simulink model "gradients_simu_v1"  (R2020b)
settings: Solver=FixedStepDiscrete  StartTime=0.0  StopTime=simTime  RelTol=1e-3
InitFcn:
  | generate_locals_for_simulink
undefined symbols (not defined in the file): gray, Hg
libraries: simulink x6, visionhdlio x3, visionhdlutilities x2, visionstatistics x1, visionhdlfilter x1, dspvision x1
settings Model: DataTypeOverride=Off  SimulationMode=accelerator  Creator=The MathWorks, Inc.  LastModifiedBy=Ethan
settings SolverCC: AutoInsertRateTranBlk=on
settings DataIOCC: LimitDataPoints=on  SaveOutput=off  SignalLogging=off  SaveTime=off  ReturnWorkspaceOutputs=off
settings OptimizationCC: BlockReduction=off  ConditionallyExecuteInputs=off  DefaultParameterBehavior=Inlined  LifeSpan=inf
settings DebuggingCC: AlgebraicLoopMsg=error  SingleTaskRateTransMsg=error  ParameterPrecisionLossMsg=none  AllowSymbolicDim=off  StrictBusMsg=ErrorOnBusTreatedAsVector  SFUnexpectedBacktrackingDiag=warning  SFNoUnconditionalDefaultTransitionDiag=warning  SFExecutionAtInitializationDiag=none  ArithmeticOperatorsInVariantConditions=warning
settings HardwareCC: ProdBitPerPointer=32  ProdBitPerSizeT=32  ProdBitPerPtrDiffT=32  ProdLargestAtomicFloat=None  ProdIntDivRoundTo=Undefined  ProdEndianess=Unspecified  ProdWordSize=32  ProdHWDeviceType=ASIC/FPGA->ASIC/FPGA  ProdEqTarget=off
settings SFSimCC: SimUseLocalCustomCode=off  CustomCodeUndefinedFunction=UseInterfaceOnly
settings RTWCC: RTWUseLocalCustomCode=off
settings CodeAppCC: StateflowObjectComments=on
settings GRTTargetCC: TargetLangStandard=C89/C90 (ANSI)
settings ConfigComp: CovMetricSettings=dw  CovSaveCumulativeToWorkspaceVar=on  CovSaveSingleToWorkspaceVar=on  CovExternalEMLEnable=off  CovSFcnEnable=off

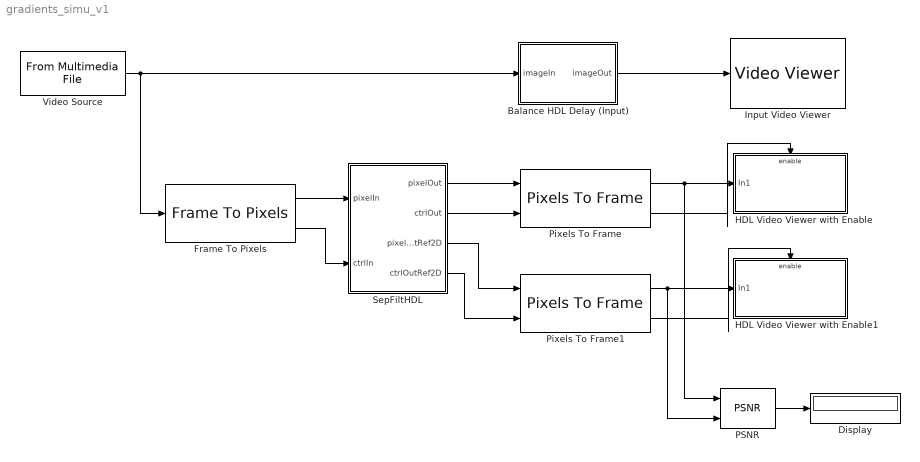
== system gradients_simu_v1 ==
  Balance HDL Delay (Input) : Subsystem
  Display : Display
  Frame To Pixels : visionhdlio/Frame To Pixels  NumComponents=1  NumPixels=1  VideoFormat=480p  ActivePixelsPerLine=32  ActiveVideoLines=18  TotalPixelsPerLine=42  TotalVideoLines=28  StartingActiveLine=6  FrontPorch=5  SampleTime=0
      settings: SourceProductName=Vision HDL Toolbox
  HDL Video Viewer with Enable : Subsystem
  HDL Video Viewer with Enable1 : Subsystem
  Input Video Viewer : VideoViewer  colormapValue=gray(256)  FigPos=[27 749 754 601]
  PSNR : visionstatistics/PSNR
      settings: SourceProductName=Computer Vision Toolbox
  Pixels To Frame : visionhdlio/Pixels To Frame  NumComponents=1  NumPixels=1  VideoFormat=480p  ActivePixelsPerLine=32  ActiveVideoLines=18  TotalPixelsPerLine=42  TotalVideoLines=28
      settings: SourceProductName=Vision HDL Toolbox
  Pixels To Frame1 : visionhdlio/Pixels To Frame  NumComponents=1  NumPixels=1  VideoFormat=480p  ActivePixelsPerLine=32  ActiveVideoLines=18  TotalPixelsPerLine=42  TotalVideoLines=28
      settings: SourceProductName=Vision HDL Toolbox
  SepFiltHDL : Subsystem
  Video Source : dspvision/From Multimedia File  inputFilename=C:\Users\Ethan\Ravven_Labs_Ethan\ravven-tag\simulink\gradients\images\start.mp4  readRange=[1 Inf]  loop=on  numPlays=inf  outputStreams=Video only  videoDataType=uint8  audioDataType=int16  inheritSampleTime=off  userDefinedSampleTime=totalPixels  noAudioOutput=off  isIntensityVideo=off  fourcc=Intensity  colorVideoFormat=One multidimensional signal  outputEOF=off  dataOrg=Column-major  audioFrameSize=1024  computeAudioFrameSize=off  outSamplingMode=Sample based
  wires:
  Frame To Pixels/1 -> SepFiltHDL/1(pixelIn)
  SepFiltHDL/1(pixelOut) -> Pixels To Frame/1
  SepFiltHDL/2(ctrlOut) -> Pixels To Frame/2
  Video Source/1 -> Frame To Pixels/1, Balance HDL Delay (Input)/1(imageIn)
  Balance HDL Delay (Input)/1(imageOut) -> Input Video Viewer/1
  Pixels To Frame/1 -> PSNR/1, HDL Video Viewer with Enable/1(In1)
  Pixels To Frame1/2 -> HDL Video Viewer with Enable1/Enable
  SepFiltHDL/3(pixelOutRef2D) -> Pixels To Frame1/1
  SepFiltHDL/4(ctrlOutRef2D) -> Pixels To Frame1/2
  Frame To Pixels/2 -> SepFiltHDL/2(ctrlIn)
  Pixels To Frame/2 -> HDL Video Viewer with Enable/Enable
  Pixels To Frame1/1 -> PSNR/2, HDL Video Viewer with Enable1/1(In1)
  PSNR/1 -> Display/1

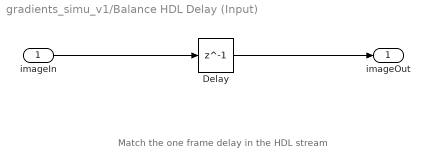
== system gradients_simu_v1/Balance HDL Delay (Input) ==
  note: Match the one frame delay in the HDL stream
  imageIn : Inport
  Delay : Delay  DelayLength=1
  imageOut : Outport  VectorParamsAs1DForOutWhenUnconnected=off
  wires:
  imageIn/1 -> Delay/1
  Delay/1 -> imageOut/1

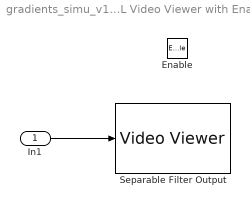
== system gradients_simu_v1/HDL Video Viewer with Enable ==
  In1 : Inport
  Enable : EnablePort
  Separable Filter Output : VideoViewer  colormapValue=gray(256)  FigPos=[579 975 702 585]
  wires:
  In1/1 -> Separable Filter Output/1

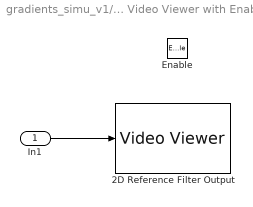
== system gradients_simu_v1/HDL Video Viewer with Enable1 ==
  In1 : Inport
  Enable : EnablePort
  2D Reference Filter Output : VideoViewer  colormapValue=gray(256)  FigPos=[1227 697 653 551]
  wires:
  In1/1 -> 2D Reference Filter Output/1

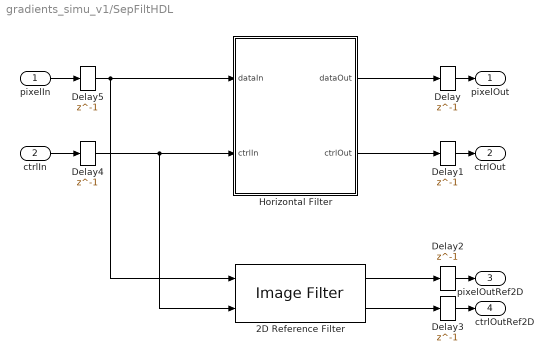
== system gradients_simu_v1/SepFiltHDL ==
  pixelIn : Inport
  ctrlIn : Inport  Port=2
  2D Reference Filter : visionhdlfilter/Image Filter  CoefficientsSource=Property  Coefficients=Hg  PaddingMethod=Constant  PaddingValue=0  LineBufferSize=2048  SimulateUsing=Code generation  roundingMode=Nearest  overflowMode=on  CoeffDataTypeStr=good_fixdt_hg  CoeffMin=[]  CoeffMax=[]  OutputMin=[]  OutputMax=[]
      settings: SourceProductName=Vision HDL Toolbox
  Delay{,1..5} (6 alike) : Delay  DelayLength=1
  Horizontal Filter : Subsystem
  pixelOut : Outport  VectorParamsAs1DForOutWhenUnconnected=off
  ctrlOut : Outport  Port=2  VectorParamsAs1DForOutWhenUnconnected=off
  pixelOutRef2D : Outport  Port=3  VectorParamsAs1DForOutWhenUnconnected=off
  ctrlOutRef2D : Outport  Port=4  VectorParamsAs1DForOutWhenUnconnected=off
  wires:
  ctrlIn/1 -> Delay4/1
  pixelIn/1 -> Delay5/1
  2D Reference Filter/2 -> Delay3/1
  2D Reference Filter/1 -> Delay2/1
  Horizontal Filter/1(dataOut) -> Delay/1
  Horizontal Filter/2(ctrlOut) -> Delay1/1
  Delay/1 -> pixelOut/1
  Delay1/1 -> ctrlOut/1
  Delay2/1 -> pixelOutRef2D/1
  Delay3/1 -> ctrlOutRef2D/1
  Delay4/1 -> Horizontal Filter/2(ctrlIn), 2D Reference Filter/2
  Delay5/1 -> Horizontal Filter/1(dataIn), 2D Reference Filter/1

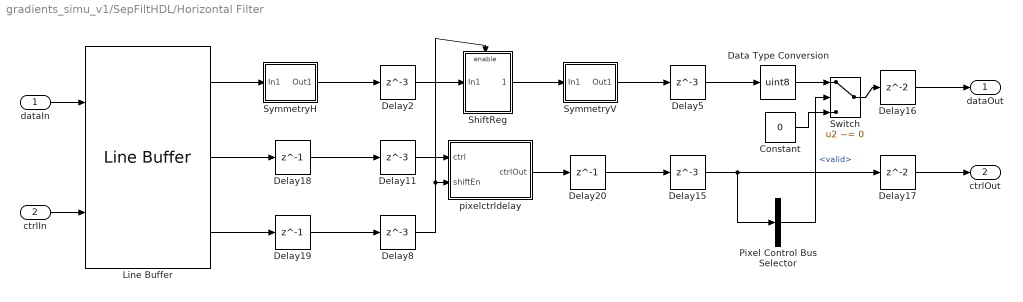
== system gradients_simu_v1/SepFiltHDL/Horizontal Filter ==
  dataIn : Inport
  ctrlIn : Inport  Port=2
  Constant : Constant  Value=0  OutDataTypeStr=Inherit: Inherit via back propagation  SampleTime=-1
  Data Type Conversion : DataTypeConversion  OutDataTypeStr=uint8  RndMeth=Nearest  SaturateOnIntegerOverflow=on
  Delay{2,5,8,11,15} (5 alike) : Delay  DelayLength=3
  Delay16 : Delay
  Delay17 : Delay
  Delay18 : Delay  DelayLength=1
  Delay19 : Delay  DelayLength=1
  Delay20 : Delay  DelayLength=1
  Line Buffer : visionhdlutilities/Line Buffer  NeighborhoodSize=[3 3]  PaddingMethod=Constant  PaddingValue=0  LineBufferSize=2048  SimulateUsing=Code generation
      settings: SourceProductName=Vision HDL Toolbox
  Pixel Control Bus Selector : BusSelector  OutputSignals=valid
  ShiftReg : Subsystem
  Switch : Switch  Criteria=u2 ~= 0
  SymmetryH : Subsystem
  SymmetryV : Subsystem
  pixelctrldelay : Subsystem
  dataOut : Outport  VectorParamsAs1DForOutWhenUnconnected=off
  ctrlOut : Outport  Port=2  VectorParamsAs1DForOutWhenUnconnected=off
  wires:
  Delay8/1 -> pixelctrldelay/2(shiftEn), ShiftReg/Enable
  SymmetryH/1(Out1) -> Delay2/1
  SymmetryV/1(Out1) -> Delay5/1
  Delay5/1 -> Data Type Conversion/1
  dataIn/1 -> Line Buffer/1
  Data Type Conversion/1 -> Switch/1
  Delay17/1 -> ctrlOut/1
  Constant/1 -> Switch/3
  Delay2/1 -> ShiftReg/1(In1)
  Switch/1 -> Delay16/1
  Delay15/1 -> Delay17/1, Pixel Control Bus Selector/1
  Pixel Control Bus Selector/1 -> Switch/2  "<valid>"
  ctrlIn/1 -> Line Buffer/2
  Delay16/1 -> dataOut/1
  Line Buffer/3 -> Delay19/1
  Line Buffer/2 -> Delay18/1
  ShiftReg/1(Out1) -> SymmetryV/1(In1)
  Line Buffer/1 -> SymmetryH/1(In1)
  Delay18/1 -> Delay11/1
  Delay19/1 -> Delay8/1
  Delay20/1 -> Delay15/1
  Delay11/1 -> pixelctrldelay/1(ctrl)
  pixelctrldelay/1(ctrlOut) -> Delay20/1

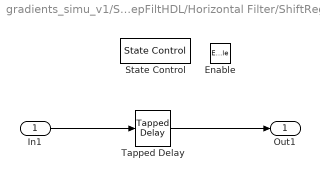
== system gradients_simu_v1/SepFiltHDL/Horizontal Filter/ShiftReg ==
  In1 : Inport
  Enable : EnablePort
  State Control : StateControl  StateControl=Synchronous
  Tapped Delay : simulink/Discrete/Tapped Delay  vinit=0.0  samptime=-1  NumDelays=3  DelayOrder=Oldest  includeCurrent=off
  Out1 : Outport  VectorParamsAs1DForOutWhenUnconnected=off
  wires:
  In1/1 -> Tapped Delay/1
  Tapped Delay/1 -> Out1/1

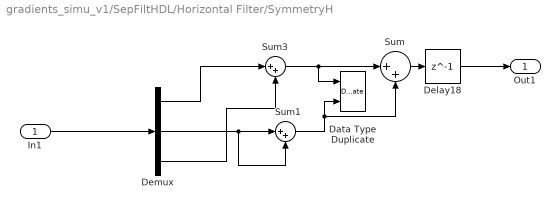
== system gradients_simu_v1/SepFiltHDL/Horizontal Filter/SymmetryH ==
  In1 : Inport
  Data Type Duplicate : DataTypeDuplicate
  Delay18 : Delay  DelayLength=1
  Demux : Demux  Outputs=3
  Sum : Sum  Inputs=|++
  Sum1 : Sum  Inputs=|++
  Sum3 : Sum  Inputs=|++
  Out1 : Outport  VectorParamsAs1DForOutWhenUnconnected=off
  wires:
  Sum3/1 -> Sum/1, Data Type Duplicate/1
  Sum1/1 -> Sum/2, Data Type Duplicate/2
  Delay18/1 -> Out1/1
  In1/1 -> Demux/1
  Demux/1 -> Sum3/1
  Demux/3 -> Sum3/2
  Demux/2 -> Sum1/2, Sum1/1
  Sum/1 -> Delay18/1

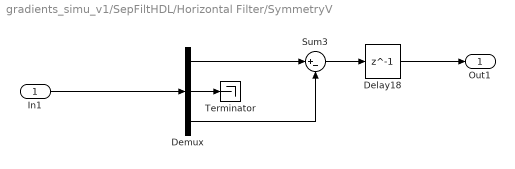
== system gradients_simu_v1/SepFiltHDL/Horizontal Filter/SymmetryV ==
  In1 : Inport
  Delay18 : Delay  DelayLength=1
  Demux : Demux  Outputs=3
  Sum3 : Sum  Inputs=|+-
  Terminator : Terminator
  Out1 : Outport  VectorParamsAs1DForOutWhenUnconnected=off
  wires:
  In1/1 -> Demux/1
  Delay18/1 -> Out1/1
  Demux/3 -> Sum3/2
  Demux/1 -> Sum3/1
  Demux/2 -> Terminator/1
  Sum3/1 -> Delay18/1

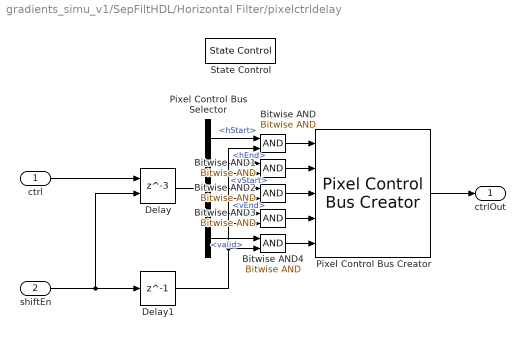
== system gradients_simu_v1/SepFiltHDL/Horizontal Filter/pixelctrldelay ==
  ctrl : Inport
  shiftEn : Inport  Port=2
  Bitwise AND{,1..4} (5 alike) : simulink/Logic and Bit Operations/Bitwise Operator  logicop=AND  UseBitMask=off  NumInputPorts=2  BitMask=bin2dec('11011001')  BitMaskRealWorld=Stored Integer
  Delay : Delay  DelayLength=3  ShowEnablePort=on
      settings: InputPortMap=u0,e6
  Delay1 : Delay  DelayLength=1
  Pixel Control Bus Creator : visionhdlutilities/Pixel Control Bus Creator
      settings: SourceProductName=Vision HDL Toolbox
  Pixel Control Bus Selector : BusSelector  OutputSignals=hStart,hEnd,vStart,vEnd,valid
  State Control : StateControl  StateControl=Synchronous
  ctrlOut : Outport  VectorParamsAs1DForOutWhenUnconnected=off
  wires:
  Bitwise AND4/1 -> Pixel Control Bus Creator/5
  Bitwise AND/1 -> Pixel Control Bus Creator/1
  Pixel Control Bus Selector/3 -> Bitwise AND2/1  "<vStart>"
  Bitwise AND3/1 -> Pixel Control Bus Creator/4
  Pixel Control Bus Selector/5 -> Bitwise AND4/1  "<valid>"
  Delay/1 -> Pixel Control Bus Selector/1
  Pixel Control Bus Selector/1 -> Bitwise AND/1  "<hStart>"
  Pixel Control Bus Selector/2 -> Bitwise AND1/1  "<hEnd>"
  Bitwise AND2/1 -> Pixel Control Bus Creator/3
  Pixel Control Bus Selector/4 -> Bitwise AND3/1  "<vEnd>"
  Bitwise AND1/1 -> Pixel Control Bus Creator/2
  Pixel Control Bus Creator/1 -> ctrlOut/1
  ctrl/1 -> Delay/1
  shiftEn/1 -> Delay1/1, Delay/2
  Delay1/1 -> Bitwise AND3/2, Bitwise AND2/2, Bitwise AND1/2, Bitwise AND/2, Bitwise AND4/2
